simulink model "target_generation_test2"  (R2016b)
settings: Solver=VariableStepAuto  StartTime=0.0  StopTime=5400  RelTol=1e-3
values from neighbouring files (symbols this model uses):
  fsw_params = init_fsw_params()    [target_generation_test_init.m]
  sc_mode = 31    [target_generation_test_init.m]
libraries: aerolibutil x4, dynamics_lib x2, GPS_time_lib x1, aerolibtransform2 x1, RW_assembly_simple_lib x1, simulink_extras x1, env_estimation_lib x1, target_generation_lib x1, command_processing x1
settings Model: Creator=Taylor  LastModifiedBy=taylorreynolds

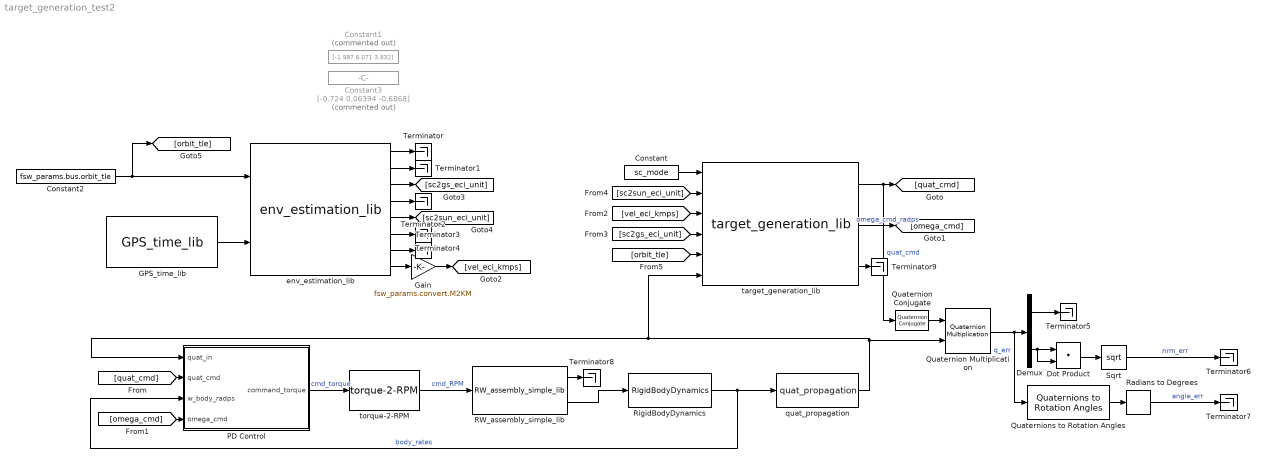
== system target_generation_test2 ==
  Constant : Constant  Value=sc_mode
  Constant1 : Constant  Commented=on  Value=[-1.987 6.071 3.832]
  Constant2 : Constant  Value=fsw_params.bus.orbit_tle
  Constant3 : Constant  Commented=on  Value=[-0.724 0.06394 -0.6868]
  Demux : Demux  Outputs=2
  Dot Product : DotProduct  InputSameDT=on  OutDataTypeStr=Inherit: Inherit via internal rule
  GPS_time_lib : GPS_time_lib/GPS_time_lib
  Gain : Gain  Gain=fsw_params.convert.M2KM
  PD Control : Subsystem  AncestorBlock=pd_control_lib/PD Control
  Quaternion Conjugate : aerolibutil/Quaternion Conjugate
  Quaternion Multiplication : aerolibutil/Quaternion Multiplication
  Quaternions to Rotation Angles : aerolibtransform2/Quaternions to Rotation Angles  rotationOrder=XYZ
  RW_assembly_simple_lib : RW_assembly_simple_lib/RW_assembly_simple_lib  natural_frequency=sim_params.actuators.reaction_wheel.natural_freq  damping_ratio=sim_params.actuators.reaction_wheel.damping  max_rate=sim_params.actuators.reaction_wheel.rate_limit
  Radians to Degrees : simulink_extras/Transformations/Radians to Degrees
  RigidBodyDynamics : dynamics_lib/Dynamics/RigidBodyDynamics
  Sqrt : Sqrt  SaturateOnIntegerOverflow=on
  Terminator{,1..9} (10 alike) : Terminator
  env_estimation_lib : env_estimation_lib/env_estimation_lib
  quat_propagation : dynamics_lib/Dynamics/quat_propagation
  target_generation_lib : target_generation_lib/target_generation_lib
  torque-2-RPM : command_processing/command_processing/torque-2-RPM
  wires:
  Constant/1 -> target_generation_lib/1
  Constant2/1 -> [orbit_tle], env_estimation_lib/1
  GPS_time_lib/1 -> env_estimation_lib/2
  RigidBodyDynamics/1 -> PD Control/3(w_body_radps), quat_propagation/1  "body_rates"
  PD Control/1(command_torque) -> torque-2-RPM/1  "cmd_torque"
  quat_propagation/1 -> target_generation_lib/6, PD Control/1(quat_in), Quaternion Multiplication/2
  env_estimation_lib/8 -> Gain/1
  target_generation_lib/1 -> Quaternion Conjugate/1, [quat_cmd]  "quat_cmd"
  target_generation_lib/2 -> [omega_cmd]  "omega_cmd_radps"
  [quat_cmd] -> PD Control/2(quat_cmd)
  [omega_cmd] -> PD Control/4(omega_cmd)
  Gain/1 -> [vel_eci_kmps]
  [vel_eci_kmps] -> target_generation_lib/3
  env_estimation_lib/1 -> Terminator/1
  env_estimation_lib/2 -> Terminator1/1
  env_estimation_lib/3 -> [sc2gs_eci_unit]
  [sc2gs_eci_unit] -> target_generation_lib/4
  env_estimation_lib/4 -> Terminator2/1
  env_estimation_lib/5 -> [sc2sun_eci_unit]
  [sc2sun_eci_unit] -> target_generation_lib/2
  env_estimation_lib/6 -> Terminator4/1
  env_estimation_lib/7 -> Terminator3/1
  [orbit_tle] -> target_generation_lib/5
  Quaternion Conjugate/1 -> Quaternion Multiplication/1
  Quaternion Multiplication/1 -> Quaternions to Rotation Angles/1, Demux/1  "q_err"
  Demux/1 -> Terminator5/1
  Demux/2 -> Dot Product/2, Dot Product/1
  Dot Product/1 -> Sqrt/1
  Sqrt/1 -> Terminator6/1  "nrm_err"
  Radians to Degrees/1 -> Terminator7/1  "angle_err"
  Quaternions to Rotation Angles/1 -> Radians to Degrees/1
  torque-2-RPM/1 -> RW_assembly_simple_lib/1  "cmd_RPM"
  RW_assembly_simple_lib/2 -> RigidBodyDynamics/1
  RW_assembly_simple_lib/1 -> Terminator8/1
  target_generation_lib/3 -> Terminator9/1

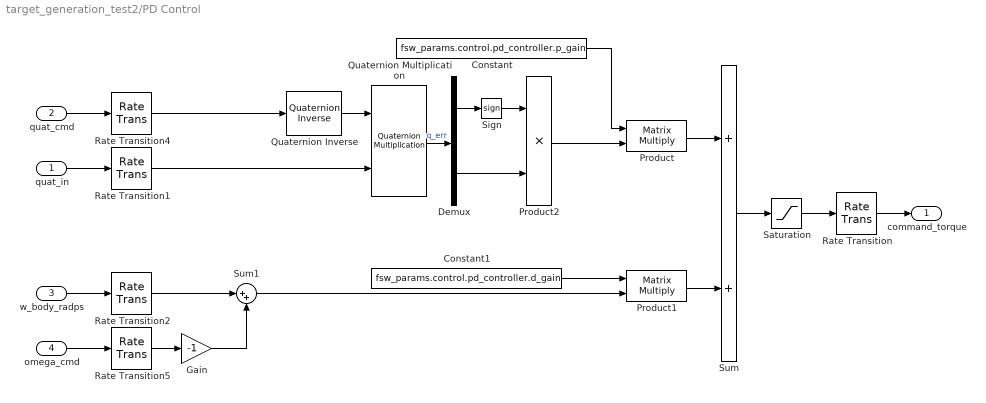
== system target_generation_test2/PD Control ==
  quat_in : Inport
  quat_cmd : Inport  Port=2
  w_body_radps : Inport  Port=3
  omega_cmd : Inport  Port=4
  Constant : Constant  Value=fsw_params.control.pd_controller.p_gain
  Constant1 : Constant  Value=fsw_params.control.pd_controller.d_gain
  Demux : Demux  Outputs=[1 3]
  Gain : Gain  Gain=-1
  Product : Product  Multiplication=Matrix(*)
  Product1 : Product  Multiplication=Matrix(*)
  Product2 : Product
  Quaternion Inverse : aerolibutil/Quaternion Inverse
  Quaternion Multiplication : aerolibutil/Quaternion Multiplication
  Rate Transition : RateTransition  X0=fsw_params.control.pd_controller.ic.rt_command_torque
  Rate Transition1 : RateTransition  X0=fsw_params.control.pd_controller.ic.rt_quat_in  OutPortSampleTime=fsw_params.control.pd_controller.sample_time_s
  Rate Transition2 : RateTransition  X0=fsw_params.control.pd_controller.ic.rt_w_body_radps  OutPortSampleTime=fsw_params.control.pd_controller.sample_time_s
  Rate Transition4 : RateTransition  X0=fsw_params.control.pd_controller.ic.rt_quat_in  OutPortSampleTime=fsw_params.control.pd_controller.sample_time_s
  Rate Transition5 : RateTransition  X0=fsw_params.control.pd_controller.ic.rt_w_body_radps  OutPortSampleTime=fsw_params.control.pd_controller.sample_time_s
  Saturation : Saturate  UpperLimit=fsw_params.control.pd_controller.max_torque  LowerLimit=-fsw_params.control.pd_controller.max_torque
  Sign : Signum
  Sum : Sum
  Sum1 : Sum  Inputs=|++
  command_torque : Outport
  wires:
  Product2/1 -> Product/2
  Sign/1 -> Product2/1
  Sum1/1 -> Product1/2
  Gain/1 -> Sum1/2
  Rate Transition5/1 -> Gain/1
  Rate Transition2/1 -> Sum1/1
  omega_cmd/1 -> Rate Transition5/1
  Rate Transition4/1 -> Quaternion Inverse/1
  Rate Transition1/1 -> Quaternion Multiplication/2
  Rate Transition/1 -> command_torque/1
  Sum/1 -> Saturation/1
  Product1/1 -> Sum/2
  Product/1 -> Sum/1
  Demux/2 -> Product2/2
  w_body_radps/1 -> Rate Transition2/1
  Demux/1 -> Sign/1
  Quaternion Multiplication/1 -> Demux/1  "q_err"
  quat_in/1 -> Rate Transition1/1
  Quaternion Inverse/1 -> Quaternion Multiplication/1
  quat_cmd/1 -> Rate Transition4/1
  Constant/1 -> Product/1
  Constant1/1 -> Product1/1
  Saturation/1 -> Rate Transition/1
